simulink model "thrustmodel"  (R2014b)
settings: Solver=FixedStepDiscrete  StartTime=0.0  StopTime=2  FixedStep=0.001  RelTol=1e-3
libraries: simulink x2
settings Model: Creator=Jostein  LastModifiedBy=Jostein

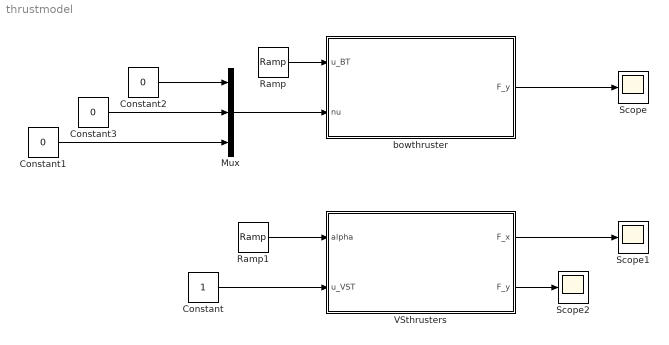
== system thrustmodel ==
  Constant : Constant
  Constant1 : Constant  Value=0
  Constant2 : Constant  Value=0
  Constant3 : Constant  Value=0
  Mux : Mux  Inputs=3
  Ramp : simulink/Sources/Ramp  slope=1  start=0  X0=-1
  Ramp1 : simulink/Sources/Ramp  slope=pi  start=0  X0=0
  Scope : Scope
      settings: TimeRange=2  YMin=-3  YMax=2
  Scope1 : Scope
  Scope2 : Scope
      settings: SaveName=ScopeData2
  VSthrusters : MATLAB Function  TreatAsAtomicUnit=on
  bowthruster : MATLAB Function  TreatAsAtomicUnit=on
  wires:
  Ramp1/1 -> VSthrusters/1(alpha)
  Constant/1 -> VSthrusters/2(u_VST)
  Ramp/1 -> bowthruster/1(u_BT)
  bowthruster/1(F_y) -> Scope/1
  VSthrusters/2(F_y) -> Scope2/1
  VSthrusters/1(F_x) -> Scope1/1
  Constant1/1 -> Mux/3
  Constant2/1 -> Mux/1
  Constant3/1 -> Mux/2
  Mux/1 -> bowthruster/2(nu)

== matlab function thrustmodel/VSthrusters ==
  data: alpha input; u_VST input; F_x output; F_y output
function [ F_x , F_y ] = fcn(alpha,u_VST)
%#codegen

% Calculating the force in x-direction
a1 =       1.107  ;
b1 =       1.001  ;
c1 =       1.564  ;
a2 =      0.3471 ;
b2 =      0.1397 ;
c2 =      -1.599  ;
a3 =      0.1558 ;
b3 =       1.993  ;
c3 =       1.886  ;
a4 =      0.1599 ;
b4 =       0.218  ;
c4 =       1.513  ;
a5 =     0.08237 ;
b5 =       2.986  ;
c5 =      -1.601  ;
a6 =     0.04641 ;
b6 =       3.964  ;
c6 =       1.738  ;

F_x =	u_VST*(	a1*sin(b1*alpha+c1) + ...
				a2*sin(b2*alpha+c2) + ...
				a3*sin(b3*alpha+c3) + ...
				a4*sin(b4*alpha+c4) + ...
				a5*sin(b5*alpha+c5) + ...
				a6*sin(b6*alpha+c6) );

% Calculating the force in y-direction
a1 =      0.7936 ;
b1 =       1.001  ;
c1 =     0.01605;
a2 =      0.2112 ;
b2 =       1.997  ;
c2 =     0.03229;
a3 =     0.07608;
b3 =       2.991  ;
c3 =       2.986  ;
a4 =     0.04817;
b4 =       3.999  ;
c4 =     -0.8668 ;
a5 =     0.01757;
b5 =       4.904  ;
c5 =      -2.622 ;
a6 =    -0.02089;
b6 =       5.068  ;
c6 =      0.2548 ;

F_y =	u_VST*(	a1*sin(b1*alpha+c1) + ...
				a2*sin(b2*alpha+c2) + ...
				a3*sin(b3*alpha+c3) + ...
				a4*sin(b4*alpha+c4) + ...
				a5*sin(b5*alpha+c5) + ...
				a6*sin(b6*alpha+c6) );

== matlab function thrustmodel/bowthruster ==
  data: u_BT input; F_y output; nu input
function F_y = fcn(u_BT,nu)
%#codegen

u = nu(1);

% Thruster characteristics
if u_BT > 0.0879
	a =       2.515;
	b =      0.1174;
	c =      -2.807;
	d =      -1.131;
	y0 = a*exp(b*u_BT) + c*exp(d*u_BT);
elseif u_BT < -0.059
	a =        -548;
	b =       0.193;
	c =       548.2;
	d =      0.1992;
	y0 = a*exp(b*u_BT) + c*exp(d*u_BT);
else
	y0 = 0;
end

% Thruster losses due to forward speed
a0 =      0.7561;
a1 =      0.3075;
b1 =      -10.22;
c1 =       2.947;

F_y = y0*(a0 + a1*atan(b1*u +c1))/1.1385;
